simulink model "inv_pend"  (R2022a)
settings: Solver=VariableStepAuto  StartTime=0.0  StopTime=100  RelTol=1e-3
values from neighbouring files (symbols this model uses):
  g = 9.81    [pendulum.m]
  J = m*L^2    (= 0.5)    [pendulum.m]
  k = 0.5    [pendulum.m]
  L = 1.0    (= 1)    [pendulum.m]
  m = 0.5    [pendulum.m]
  Ts = 0.1    [pendulum.m]
undefined symbols (not defined in the file or in its folder): DiscIntNeverNeededParam, K
settings Model: Creator=Admin  LastModifiedBy=Admin

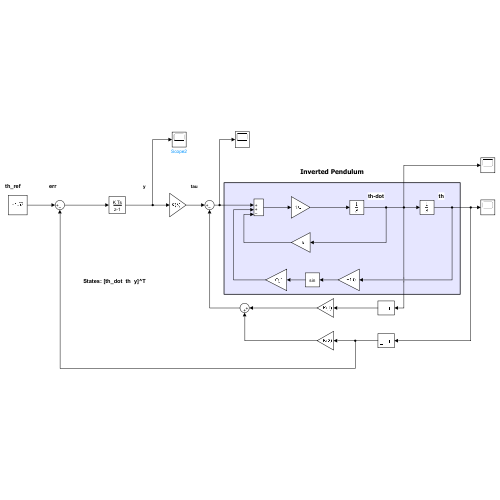
[thumbnail: Simulink's stored preview of the top-level diagram]
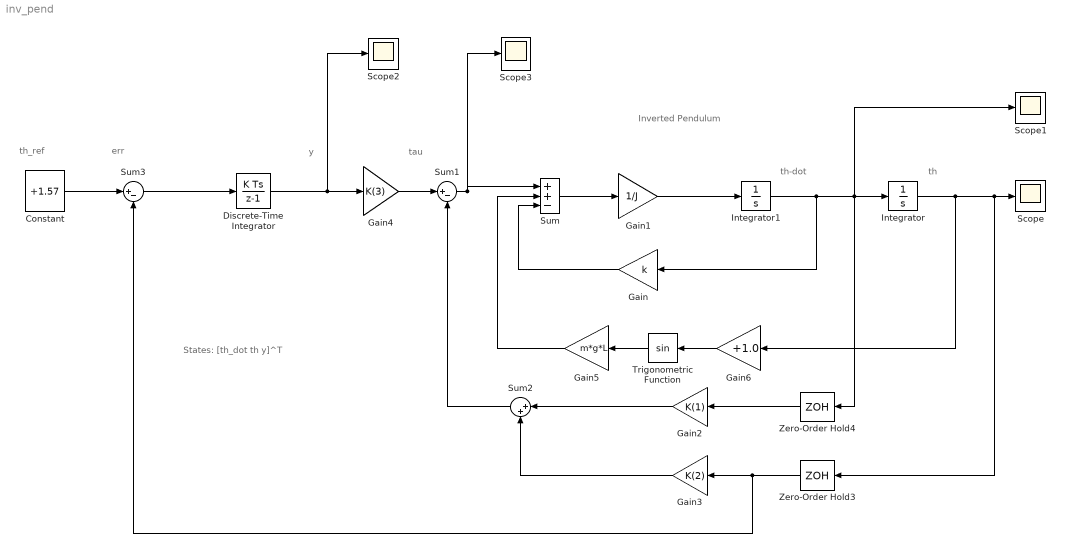
== system inv_pend ==
  note: States: [th_dot th y]^T
  note: Inverted Pendulum
  note: th
  note: th-dot
  note: tau
  note: th_ref
  note: err
  note: y
  Constant : Constant  Value=+1.57  SampleTime=Ts
  Discrete-Time Integrator : DiscreteIntegrator  gainval=1  SampleTime=-1  ICPrevOutput=DiscIntNeverNeededParam  ICPrevScaledInput=DiscIntNeverNeededParam
  Gain : Gain  Gain=k
  Gain1 : Gain  Gain=1/J
  Gain2 : Gain  Gain=K(1)
  Gain3 : Gain  Gain=K(2)
  Gain4 : Gain  Gain=K(3)
  Gain5 : Gain  Gain=m*g*L
  Gain6 : Gain  Gain=+1.0
  Integrator : Integrator  InitialCondition=0.0
  Integrator1 : Integrator
  Scope{,1..3} (4 alike) : Scope
  Sum : Sum  Inputs=|++-
  Sum1 : Sum  Inputs=|+-
  Sum2 : Sum  Inputs=|++
  Sum3 : Sum  Inputs=|+-
  Trigonometric Function : Trigonometry
  Zero-Order Hold3 : ZeroOrderHold  SampleTime=Ts
  Zero-Order Hold4 : ZeroOrderHold  SampleTime=Ts
  wires:
  Sum/1 -> Gain1/1
  Sum1/1 -> Scope3/1, Sum/1
  Gain2/1 -> Sum2/1
  Integrator/1 -> Gain6/1, Zero-Order Hold3/1, Scope/1
  Integrator1/1 -> Gain/1, Zero-Order Hold4/1, Scope1/1, Integrator/1
  Gain1/1 -> Integrator1/1
  Gain4/1 -> Sum1/1
  Discrete-Time Integrator/1 -> Gain4/1, Scope2/1
  Trigonometric Function/1 -> Gain5/1
  Gain/1 -> Sum/3
  Gain5/1 -> Sum/2
  Constant/1 -> Sum3/1
  Zero-Order Hold3/1 -> Gain3/1, Sum3/2
  Zero-Order Hold4/1 -> Gain2/1
  Gain3/1 -> Sum2/2
  Sum3/1 -> Discrete-Time Integrator/1
  Sum2/1 -> Sum1/2
  Gain6/1 -> Trigonometric Function/1
